simulink model "SOCMAIN1"  (R2024b)
settings: Solver=VariableStepAuto  StartTime=0.0  StopTime=62000  RelTol=1e-3
undefined symbols (not defined in the file): Ion, Lithium
libraries: spsIdealSwitchLib x4, spsSeriesRLCLoadLib x2, spsBatteryLib x1, spsDCVoltageSourceLib x1, sps_lib x1
settings Model: PacingRate=4  Creator=saive  LastModifiedBy=saive

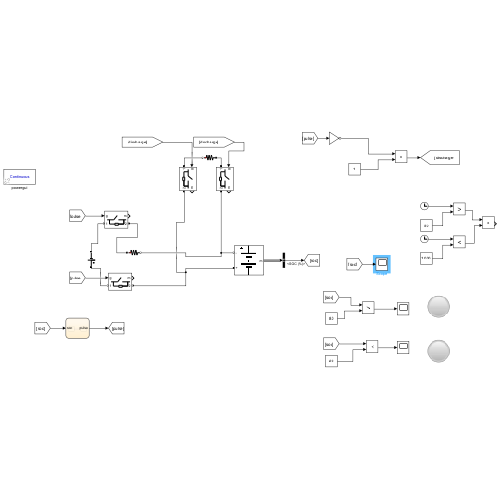
[thumbnail: Simulink's stored preview of the top-level diagram]
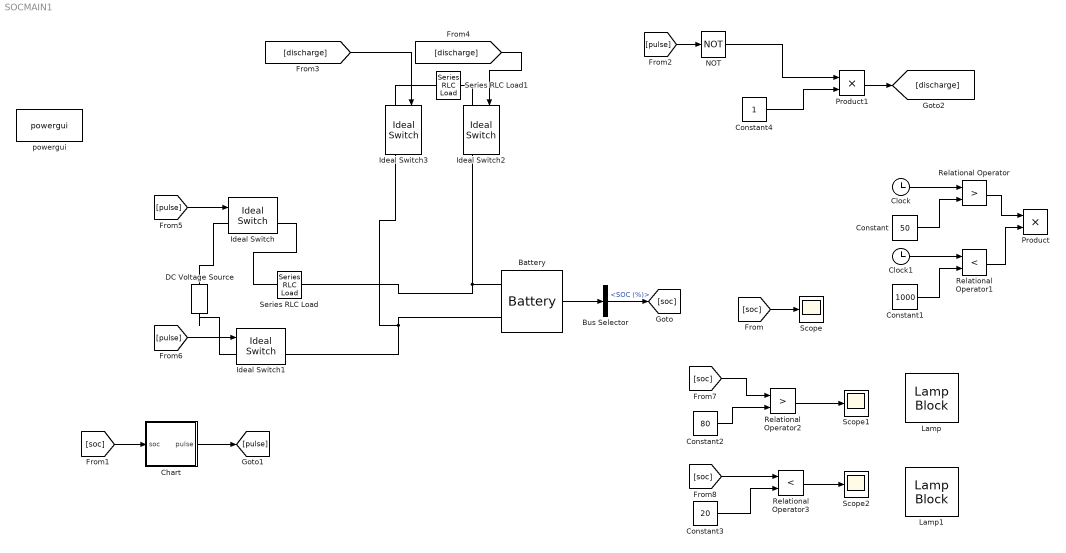
== system SOCMAIN1 ==
  Battery : spsBatteryLib/Battery  BatType=Lithium-Ion  NomV=3.85  NomQ=4  SOC=0  Batt_Tr=30  PresetModel=on  MaxQ=4  MinV=2.8875  FullV=4.4814  Dis_rate=1.7391  R=0.009625  Normal_OP=3.6174  expZone="[4.1595     0.19652]"
  Bus Selector : BusSelector  OutputSignals=SOC (%)
  Chart : Stateflow chart  TreatAsAtomicUnit=on
  Clock : Clock
  Clock1 : Clock
  Constant : Constant  Value=50
  Constant1 : Constant  Value=1000
  Constant2 : Constant  Value=80
  Constant3 : Constant  Value=20
  Constant4 : Constant
  DC Voltage Source : spsDCVoltageSourceLib/DC Voltage Source  Amplitude=15  Measurements=None
  Ideal Switch{,1..3} (4 alike) : spsIdealSwitchLib/Ideal Switch  Ron=0.001  Lon=0  IC=0  Rs=1e5  Cs=inf  Measurements=on
  Lamp : LampBlock  LabelPosition=Hide
  Lamp1 : LampBlock  LabelPosition=Hide
  NOT : Logic  Operator=NOT  IconShape=distinctive  AllPortsSameDT=off  OutDataTypeStr=boolean
  Product : Product
  Product1 : Product
  Relational Operator : RelationalOperator  Operator=>  OutDataTypeStr=boolean  RndMeth=Simplest  InputSameDT=off
  Relational Operator1 : RelationalOperator  Operator=<  OutDataTypeStr=boolean  RndMeth=Simplest  InputSameDT=off
  Relational Operator2 : RelationalOperator  Operator=>  OutDataTypeStr=boolean  RndMeth=Simplest  InputSameDT=off
  Relational Operator3 : RelationalOperator  Operator=<  OutDataTypeStr=boolean  RndMeth=Simplest  InputSameDT=off
  Scope : Scope
  Scope1 : Scope
  Scope2 : Scope
  Series RLC Load : spsSeriesRLCLoadLib/Series RLC Load  LConnTagsString=a  RConnTagsString=__new0  NominalVoltage=10  NominalFrequency=60  ActivePower=1000  InductivePower=00  CapacitivePower=0  Setx0=off  InitialVoltage=0  SetiL0=off  InitialCurrent=0  Measurements=None  LoadType=constant Z
  Series RLC Load1 : spsSeriesRLCLoadLib/Series RLC Load  LConnTagsString=a  RConnTagsString=__new0  NominalVoltage=10  NominalFrequency=60  ActivePower=3.5  InductivePower=00  CapacitivePower=0  Setx0=off  InitialVoltage=0  SetiL0=off  InitialCurrent=0  Measurements=None  LoadType=constant Z
  powergui : sps_lib/powergui  Priority=1  SimulationMode=Continuous  SampleTime=50e-6  frequency=60  Iterations=50  frequencyindice=0  Pbase=100e6  ErrMax=1e-4  UnitsV=kV  UnitsW=MW  buscounter=0  FunctionMessages=off  echomessages=off  EnableUseOfTLC=off  CurrentSourceSwitches=off  DisableSnubberDevices=off  DisableRonSwitches=off  DisableVfSwitches=off  DisplayEquations=off  AutomaticDiscreteSolvers=off  SolverType=Tustin/Backward Euler (TBE)  Interpol=off  ExternalGateDelay=off  methode=off  Ts=100  x0status=blocks  SPID=on  SwTol=0  HookPort=off  NonlinearTolerance=1e-4  nMaxIteration=100  ContinueOnMaxIteration=off  RestoreLinks=warning  ResistiveCurrentMeasurement=off  Frange=[0:2:500]  Ylog=off  Xlog=on  ShowGrid=off  save=off  variable=ZData  structure=0  ZoomFFT=off  StartTime=0.0  cycles=1  DisplayStyle=1  fundamental=60  FreqAxis=off  MaxFrequency=1000  frequencyindicesteady=1  RmsSteady=1  display=off
  wires:
  Battery/1 -> Bus Selector/1
  Bus Selector/1 -> [soc]  "<SOC (%)>"
  [soc] -> Scope/1
  Clock/1 -> Relational Operator/1
  Constant/1 -> Relational Operator/2
  Constant1/1 -> Relational Operator1/2
  Clock1/1 -> Relational Operator1/1
  [pulse] -> NOT/1
  Relational Operator/1 -> Product/1
  Relational Operator1/1 -> Product/2
  NOT/1 -> Product1/1
  Product1/1 -> [discharge]
  [discharge] -> Ideal Switch2/1
  [discharge] -> Ideal Switch3/1
  [soc] -> Chart/1(soc)
  Chart/1(pulse) -> [pulse]
  [pulse] -> Ideal Switch1/1
  [pulse] -> Ideal Switch/1
  [soc] -> Relational Operator2/1
  Constant2/1 -> Relational Operator2/2
  Relational Operator2/1 -> Scope1/1
  Relational Operator3/1 -> Scope2/1
  [soc] -> Relational Operator3/1
  Constant3/1 -> Relational Operator3/2
  Constant4/1 -> Product1/2
  connections:
  Ideal Switch1/RConn1 -- Battery/LConn1 -- Ideal Switch3/RConn1
  DC Voltage Source/LConn1 -- Ideal Switch/LConn1
  Series RLC Load/RConn1 -- Ideal Switch2/RConn1 -- Battery/LConn2
  DC Voltage Source/RConn1 -- Ideal Switch1/LConn1
  Ideal Switch/RConn1 -- Series RLC Load/LConn1
  Series RLC Load1/LConn1 -- Ideal Switch3/LConn1
  Series RLC Load1/RConn1 -- Ideal Switch2/LConn1

== stateflow chart SOCMAIN1/Chart ==
  state dharge
    entry : pulse =1
  state discharge
    entry : pulse =0
  (default) -> dharge
  dharge -> discharge : [soc>80]
  discharge -> dharge : [soc<20
      |
      | ]
  data: soc input; pulse output
